simulink model "HT07CombinedPowertrainThermalModelv2IsolatedMotors"  (R2022b)
settings: Solver=VariableStepAuto  StartTime=0.0  StopTime=timeEnd  RelTol=1e-4
values from neighbouring files (symbols this model uses):
  Tamb = 26    [HT07CombinedPowertrainThermalSetupExperimental.m]
undefined symbols (not defined in the file or in its folder): AH, convectionArea, DiscIntNeverNeededParam, radiator, SOC0, startTempC, tabResis
libraries: fl_lib x161, nesl_utility x41, SimscapeFluids_lib x16, ee_lib x2
(part 5 of 5)

== system HT07CombinedPowertrainThermalModelv2IsolatedMotors/Accumulator/SOC Calculation ==
  I [A] : Inport
  1/(nominal battery capacity) : Gain  Gain=1/(AH*3600)
  Discrete-Time Integrator : DiscreteIntegrator  SampleTime=-1  ICPrevOutput=DiscIntNeverNeededParam  ICPrevScaledInput=DiscIntNeverNeededParam
  Initial State of Charge : Constant  Value=SOC0
  Multiply : Gain
  Rate Transition2 : RateTransition
  Sum2 : Sum  Inputs=+-
  SOC [0,1] : Outport  VectorParamsAs1DForOutWhenUnconnected=off
  wires:
  Rate Transition2/1 -> 1/(nominal battery capacity)/1
  1/(nominal battery capacity)/1 -> Discrete-Time Integrator/1
  Initial State of Charge/1 -> Sum2/1
  Discrete-Time Integrator/1 -> Sum2/2
  Sum2/1 -> SOC [0,1]/1
  I [A]/1 -> Multiply/1
  Multiply/1 -> Rate Transition2/1
